simulink model "eCS_Algo_Simulation_2015b"  (R2015b)
settings: Solver=ode1  StartTime=0.0  StopTime=3  FixedStep=1/80000  RelTol=1e-3
PreLoadFcn:
  | if exist('tl_preloadfcn','file'), tl_preloadfcn(gcs,402); end
PostLoadFcn:
  | , if any(exist('dsrtsu_mdlpostloadfcn', 'file') == [2, 3, 6]), try dsrtsu_mdlpostloadfcn('Execute', bdroot); catch fprintf('Error in PostLoadFcn (dsrtsu_mdlpostloadfcn) for model "%s":\n %s\n', bdroot, lasterr); end, end,
  | if exist('tl_postloadfcn','file'), tl_postloadfcn(gcs,402); end
InitFcn:
  | Omegan=1.3024e+03;
  | xi=0.9; %0.48
  | K=0.1931;
  | K1=0.0198;
  | TauLocked=0.00255;
  | TauUnLocked=0.0042;
  | Kp=1/(2*K1);
  | Ki=Kp/((TauLocked+TauUnLocked)/2);
  | if exist('tlds_init','file'), tlds_init(gcs); end
StartFcn:
  | if exist('tlds_start','file'), tlds_start(gcs); end
StopFcn:
  | if exist('tlds_stop','file'), tlds_stop(gcs); end
model workspace (MAT data in the model file):
  au8PrevExecProfile = [0 0 0 0 0 0]
values from neighbouring files (symbols this model uses):
  AccSensor = 5    [Parameter_eCS_Algo.m]
  AlgoType = 0    [Parameter_eCS_Algo.m]
  Cxy = 1*0.017    (= 0.017)    [Acc_Init_SelV1.m]
  Cxz = 1*0.017    (= 0.017)    [Acc_Init_SelV1.m]
  Cyx = 1*0.017    (= 0.017)    [Acc_Init_SelV1.m]
  Cyz = 1*0.017    (= 0.017)    [Acc_Init_SelV1.m]
  Czx = 1*0.017    (= 0.017)    [Acc_Init_SelV1.m]
  Czy = 1*0.017    (= 0.017)    [Acc_Init_SelV1.m]
  Forced_Oscillation = 0    [Parameter_eCS_Algo.m]    (also in run_Rotation_sim.m = run)
  FreqTemperature = 10    [Acc_Init_SelV1.m]
  MaxSensorOffset = 0.3    [Acc_Init_SelV1.m]
  Mean_x_noise = 4e-3    (= 0.004)    [Acc_Init_SelV1.m]
  Mean_y_noise = 4e-3    (= 0.004)    [Acc_Init_SelV1.m]
  Mean_z_noise = 4e-3    (= 0.004)    [Acc_Init_SelV1.m]
  ODR = 8000    [Acc_Init_SelV1.m]
  offsetcorrection_on_off = 0    [Parameter_eCS_Algo.m]
  phi_pulse_rotation = 0    [Parameter_eCS_Algo.m]    (also in run_Rotation_sim.m = angle)
  pulsetype = 2    [Parameter_eCS_Algo.m]    (also in run_simulation.m = j; run_simulation_ActiveX.m = j)
  Range = 4    [Acc_Init_SelV1.m]
  sensitivity_optimisation = 0    [Parameter_eCS_Algo.m]
  TempBias = 0    [Acc_Init_SelV1.m]
  TemperatureAmp = 0    [Acc_Init_SelV1.m]
  Var_x_noise = 1.84e-9    (= 1.84e-09)    [Acc_Init_SelV1.m]
  Var_y_noise = 2.025e-09    [Acc_Init_SelV1.m]
  Var_z_noise = 1.374e-09    [Acc_Init_SelV1.m]
  w_x = 2*pi*F_x    (= 376.991118431)    [Acc_Init_SelV1.m]
  w_y = 2*pi*F_y    (= 376.991118431)    [Acc_Init_SelV1.m]
  w_z = 2*pi*F_z    (= 376.991118431)    [Acc_Init_SelV1.m]
  x_max_temp_drift = 0.061    [Acc_Init_SelV1.m]
  x_offset_enable = 0    [Acc_Init_SelV1.m]
  x_run_to_run_drift = 0.0    (= 0)    [Acc_Init_SelV1.m]
  x_temp_co_drift = 0.000    (= 0)    [Acc_Init_SelV1.m]
  Xi_x = 0.7    [Acc_Init_SelV1.m]
  Xi_y = 0.7    [Acc_Init_SelV1.m]
  Xi_z = 0.7    [Acc_Init_SelV1.m]
  y_max_temp_drift = 0.061    [Acc_Init_SelV1.m]
  y_offset_enable = 0    [Acc_Init_SelV1.m]
  y_run_to_run_drift = 0.0    (= 0)    [Acc_Init_SelV1.m]
  y_temp_co_drift = 0.000    (= 0)    [Acc_Init_SelV1.m]
  z_max_temp_drift = 0.13    [Acc_Init_SelV1.m]
  z_offset_enable = 0    [Acc_Init_SelV1.m]
  z_run_to_run_drift = 0.0    (= 0)    [Acc_Init_SelV1.m]
  z_temp_co_drift = 0.000    (= 0)    [Acc_Init_SelV1.m]
undefined symbols (not defined in the file or in its folder): controller_sample_rate, ddv, DiscIntNeverNeededParam, gmw_roada_x__m_s__, gmw_roada_y__m_s__, gmw_roadtime_2kHz, KSF_50_a_x, KSF_50_a_y, KSF_50_time, KSG_30_a_x, KSG_30_a_y, KSG_30_time, Meldorf_HindenburgstraAcceleration_x__m_s_2_, Meldorf_HindenburgstraAcceleration_y__m_s_2_, Meldorf_HindenburgstraAcceleration_z__m_s_2_, Meldorf_HindenburgstraTime__s_, pulse_FF27, pulse_MPDB, pulse_ODB40, pulse_ODB64, pulse_USNCAP, pulsetime_FF27, pulsetime_MPDB, pulsetime_ODB40, pulsetime_ODB64, pulsetime_USNCAP, Rauasphalt_60_a_x, Rauasphalt_60_a_y, Rauasphalt_60_time, sigbuilder_block, VW_416_2kHza_x_2kHz, VW_416_2kHza_y_2kHz, VW_416_2kHztime_2kHz
libraries: simulink x29, tllib x23, tl_autosar_lib x15, simulink_extras x7, LIB_TF_G_111 x2, LIB_TF_G_12_StepControl x2, LIB_TF_G_112 x1, dspsigops x1
(part 6 of 13)

== system eCS_Algo_Simulation_2015b/SAD/Subsystem/SAD/SAD/SAD_Init/For ==
  Assignment : Assignment  IndexMode=Zero-based  IndexOptions=Index vector (port)  Indices=1  OutputSizes=1  mask(TL_Assignment){data={'insideiteratedsystem',logical(1),'omitinitializations',1,'output',{'variable','SAD/Vars/au8FollowingCycle','inheritscaling',0},'date',738430.41690026619}}
      settings: CopyFcn=if exist('tl_reset_reviewflag') == 2, tl_reset_reviewflag(gcbh); end  DeleteFcn=if exist('delete_tlblock','file')==2,delete_tlblock(gcbh);end  NameChangeFcn=if exist('rename_tlblock','file')==2,rename_tlblock(gcbh);end  OpenFcn=if exist('tl_open_blockdlg','file')==2,tl_open_blockdlg(gcbh);else,open_system(gcbh,'parameter');end
      mask Help: eval(['if exist(''tl_online_help'',''file'') == 2, tl_online_help(''Topic'',''TL_Assignment''),else, web([''jar:file:///'',matlabroot,''/help/toolbox/simulink/help.jar!/slref/' lower(get_param(gcbh,'Blocktype')) '.html''], ''-helpbrowser''),end'])
      mask Display: plot([-0.1, 1.05, NaN, -0.1, 1.05],[.01, .01, NaN, .99, .99]);
  BusCreator : BusCreator  Inputs=2
  Constant : Constant  Value=[255 255 255 255]  mask(TL_Constant){data={'date',738430.41690041672}}
      settings: CopyFcn=if exist('tl_reset_reviewflag','file')==2,tl_reset_reviewflag(gcbh);end  DeleteFcn=if exist('delete_tlblock','file')==2,delete_tlblock(gcbh);end  NameChangeFcn=if exist('rename_tlblock','file')==2,rename_tlblock(gcbh);end  OpenFcn=if exist('tl_open_blockdlg','file')==2,tl_open_blockdlg(gcbh);else,open_system(gcbh,'parameter');end
      mask Help: eval(['if exist(''tl_online_help'',''file'') == 2, tl_online_help(''Topic'',''TL_Constant''),else, web([''jar:file:///'',matlabroot,''/help/toolbox/simulink/help.jar!/slref/' lower(get_param(gcbh,'Blocktype')) '.html''], ''-helpbrowser''),end'])
      mask Display: plot([-0.1, 1.05, NaN, -0.1, 1.05],[.01, .01, NaN, .99, .99]);
  Constant1 : Constant  Value=ddv('SAD/Macros/Profiles/KU8_PROFILE_SIZE')  mask(TL_Constant){data={'output',{'variable','SAD/Macros/Profiles/KU8_PROFILE_SIZE'},'date',738430.41690053244}}
      settings: CopyFcn=if exist('tl_reset_reviewflag','file')==2,tl_reset_reviewflag(gcbh);end  DeleteFcn=if exist('delete_tlblock','file')==2,delete_tlblock(gcbh);end  NameChangeFcn=if exist('rename_tlblock','file')==2,rename_tlblock(gcbh);end  OpenFcn=if exist('tl_open_blockdlg','file')==2,tl_open_blockdlg(gcbh);else,open_system(gcbh,'parameter');end
      mask Help: eval(['if exist(''tl_online_help'',''file'') == 2, tl_online_help(''Topic'',''TL_Constant''),else, web([''jar:file:///'',matlabroot,''/help/toolbox/simulink/help.jar!/slref/' lower(get_param(gcbh,'Blocktype')) '.html''], ''-helpbrowser''),end'])
      mask Display: plot([-0.1, 1.05, NaN, -0.1, 1.05],[.01, .01, NaN, .99, .99]);
  Constant2 : Constant  Value=[255 255 255 255]  mask(TL_Constant){data={'date',738430.41690065968}}
      settings: CopyFcn=if exist('tl_reset_reviewflag','file')==2,tl_reset_reviewflag(gcbh);end  DeleteFcn=if exist('delete_tlblock','file')==2,delete_tlblock(gcbh);end  NameChangeFcn=if exist('rename_tlblock','file')==2,rename_tlblock(gcbh);end  OpenFcn=if exist('tl_open_blockdlg','file')==2,tl_open_blockdlg(gcbh);else,open_system(gcbh,'parameter');end
      mask Help: eval(['if exist(''tl_online_help'',''file'') == 2, tl_online_help(''Topic'',''TL_Constant''),else, web([''jar:file:///'',matlabroot,''/help/toolbox/simulink/help.jar!/slref/' lower(get_param(gcbh,'Blocktype')) '.html''], ''-helpbrowser''),end'])
      mask Display: plot([-0.1, 1.05, NaN, -0.1, 1.05],[.01, .01, NaN, .99, .99]);
  Constant3 : Constant  Value=ddv('Common/KU8_THREE')  mask(TL_Constant){data={'output',{'variable','Common/KU8_THREE'},'date',738430.41690077551}}
      settings: CopyFcn=if exist('tl_reset_reviewflag','file')==2,tl_reset_reviewflag(gcbh);end  DeleteFcn=if exist('delete_tlblock','file')==2,delete_tlblock(gcbh);end  NameChangeFcn=if exist('rename_tlblock','file')==2,rename_tlblock(gcbh);end  OpenFcn=if exist('tl_open_blockdlg','file')==2,tl_open_blockdlg(gcbh);else,open_system(gcbh,'parameter');end
      mask Help: eval(['if exist(''tl_online_help'',''file'') == 2, tl_online_help(''Topic'',''TL_Constant''),else, web([''jar:file:///'',matlabroot,''/help/toolbox/simulink/help.jar!/slref/' lower(get_param(gcbh,'Blocktype')) '.html''], ''-helpbrowser''),end'])
      mask Display: plot([-0.1, 1.05, NaN, -0.1, 1.05],[.01, .01, NaN, .99, .99]);
  Constant4 : Constant  Value=ddv('SAD/NVP/Profiles/CFG_au8ProfileLib')  mask(TL_Constant){data={'output',{'variable','SAD/NVP/Profiles/CFG_au8ProfileLib'},'date',738430.41690089123}}
      settings: CopyFcn=if exist('tl_reset_reviewflag','file')==2,tl_reset_reviewflag(gcbh);end  DeleteFcn=if exist('delete_tlblock','file')==2,delete_tlblock(gcbh);end  NameChangeFcn=if exist('rename_tlblock','file')==2,rename_tlblock(gcbh);end  OpenFcn=if exist('tl_open_blockdlg','file')==2,tl_open_blockdlg(gcbh);else,open_system(gcbh,'parameter');end
      mask Help: eval(['if exist(''tl_online_help'',''file'') == 2, tl_online_help(''Topic'',''TL_Constant''),else, web([''jar:file:///'',matlabroot,''/help/toolbox/simulink/help.jar!/slref/' lower(get_param(gcbh,'Blocktype')) '.html''], ''-helpbrowser''),end'])
      mask Display: plot([-0.1, 1.05, NaN, -0.1, 1.05],[.01, .01, NaN, .99, .99]);
  Constant5 : Constant  mask(TL_Constant){data={'date',738430.41690100695}}
      settings: CopyFcn=if exist('tl_reset_reviewflag') == 2, tl_reset_reviewflag(gcbh); end  DeleteFcn=if exist('delete_tlblock','file')==2,delete_tlblock(gcbh);end  NameChangeFcn=if exist('rename_tlblock','file')==2,rename_tlblock(gcbh);end  OpenFcn=if exist('tl_open_blockdlg','file')==2,tl_open_blockdlg(gcbh);else,open_system(gcbh,'parameter');end
      mask Help: eval(['if exist(''tl_online_help'',''file'') == 2, tl_online_help(''Topic'',''TL_Constant''),else, web([''jar:file:///'',matlabroot,''/help/toolbox/simulink/help.jar!/slref/' lower(get_param(gcbh,'Blocktype')) '.html''], ''-helpbrowser''),end'])
      mask Display: plot([-0.1, 1.05, NaN, -0.1, 1.05],[.01, .01, NaN, .99, .99]);
  FollowingCycle : Selector  IndexMode=Zero-based  IndexOptions=Index vector (port)  Indices=[1 3]  OutputSizes=1
  For Iterator : ForIterator  IterationLimit=4  IndexMode=Zero-based  IterationVariableDataType=int8
  Product1 : Product  Inputs=**  RndMeth=Zero  mask(TL_Product){data={'output',{'type','UInt16'},'date',738430.41690100695}}
      settings: CopyFcn=if exist('tl_reset_reviewflag') == 2, tl_reset_reviewflag(gcbh); end  DeleteFcn=if exist('delete_tlblock','file')==2,delete_tlblock(gcbh);end  NameChangeFcn=if exist('rename_tlblock','file')==2,rename_tlblock(gcbh);end  OpenFcn=if exist('tl_open_blockdlg','file')==2,tl_open_blockdlg(gcbh);else,open_system(gcbh,'parameter');end
      mask Help: eval(['if exist(''tl_online_help'',''file'') == 2, tl_online_help(''Topic'',''TL_Product''),else, web([''jar:file:///'',matlabroot,''/help/toolbox/simulink/help.jar!/slref/' lower(get_param(gcbh,'Blocktype')) '.html''], ''-helpbrowser''),end'])
      mask Display: plot([-0.1, 1.05, NaN, -0.1, 1.05],[.01, .01, NaN, .99, .99]);
  Rescaler : DataTypeConversion  mask(TL_Rescaler){data={'output',{'type','UInt8'},'date',738430.4169011343}}
      settings: DeleteFcn=if exist('delete_tlblock','file')==2,delete_tlblock(gcbh);end  NameChangeFcn=if exist('rename_tlblock','file')==2,rename_tlblock(gcbh);end  OpenFcn=if exist('tl_open_blockdlg','file')==2,tl_open_blockdlg(gcbh);else,open_system(gcbh,'parameter');end
      mask Help: eval(['if exist(''tl_online_help'',''file'') == 2, tl_online_help(''Topic'',''TL_Rescaler''),else, web([''jar:file:///'',matlabroot,''/help/toolbox/simulink/help.jar!/slref/' lower(get_param(gcbh,'Blocktype')) '.html''], ''-helpbrowser''),end'])
      mask Display: plot([-0.1, 1.05, NaN, -0.1, 1.05],[.01, .01, NaN, .99, .99]);
  Rescaler1 : DataTypeConversion  mask(TL_Rescaler){data={'output',{'type','UInt8'},'date',738430.41690125002}}
      settings: DeleteFcn=if exist('delete_tlblock','file')==2,delete_tlblock(gcbh);end  NameChangeFcn=if exist('rename_tlblock','file')==2,rename_tlblock(gcbh);end  OpenFcn=if exist('tl_open_blockdlg','file')==2,tl_open_blockdlg(gcbh);else,open_system(gcbh,'parameter');end
      mask Help: eval(['if exist(''tl_online_help'',''file'') == 2, tl_online_help(''Topic'',''TL_Rescaler''),else, web([''jar:file:///'',matlabroot,''/help/toolbox/simulink/help.jar!/slref/' lower(get_param(gcbh,'Blocktype')) '.html''], ''-helpbrowser''),end'])
      mask Display: plot([-0.1, 1.05, NaN, -0.1, 1.05],[.01, .01, NaN, .99, .99]);
  Sum : Sum  mask(TL_Sum){data={'output',{'type','UInt16'},'date',738430.41690136574}}
      settings: CopyFcn=if exist('tl_reset_reviewflag') == 2, tl_reset_reviewflag(gcbh); end  DeleteFcn=if exist('delete_tlblock','file')==2,delete_tlblock(gcbh);end  NameChangeFcn=if exist('rename_tlblock','file')==2,rename_tlblock(gcbh);end  OpenFcn=if exist('tl_open_blockdlg','file')==2,tl_open_blockdlg(gcbh);else,open_system(gcbh,'parameter');end
      mask Help: eval(['if exist(''tl_online_help'',''file'') == 2, tl_online_help(''Topic'',''TL_Sum''),else, web([''jar:file:///'',matlabroot,''/help/toolbox/simulink/help.jar!/slref/' lower(get_param(gcbh,'Blocktype')) '.html''], ''-helpbrowser''),end'])
      mask Display: plot([-0.1, 1.05, NaN, -0.1, 1.05],[.01, .01, NaN, .99, .99]);
  Sum2 : Sum  Inputs=+-  mask(TL_Sum){data={'output',{'type','UInt8'},'date',738430.41690148145}}
      settings: CopyFcn=if exist('tl_reset_reviewflag') == 2, tl_reset_reviewflag(gcbh); end  DeleteFcn=if exist('delete_tlblock','file')==2,delete_tlblock(gcbh);end  NameChangeFcn=if exist('rename_tlblock','file')==2,rename_tlblock(gcbh);end  OpenFcn=if exist('tl_open_blockdlg','file')==2,tl_open_blockdlg(gcbh);else,open_system(gcbh,'parameter');end
      mask Help: eval(['if exist(''tl_online_help'',''file'') == 2, tl_online_help(''Topic'',''TL_Sum''),else, web([''jar:file:///'',matlabroot,''/help/toolbox/simulink/help.jar!/slref/' lower(get_param(gcbh,'Blocktype')) '.html''], ''-helpbrowser''),end'])
      mask Display: plot([-0.1, 1.05, NaN, -0.1, 1.05],[.01, .01, NaN, .99, .99]);
  Switch : Switch  Criteria=u2 ~= 0  mask(TL_Switch){data={'output',{'type','UInt8'},'date',738430.41690159717}}
      settings: CopyFcn=if exist('tl_reset_reviewflag') == 2, tl_reset_reviewflag(gcbh); end  DeleteFcn=if exist('delete_tlblock','file')==2,delete_tlblock(gcbh);end  NameChangeFcn=if exist('rename_tlblock','file')==2,rename_tlblock(gcbh);end  OpenFcn=if exist('tl_open_blockdlg','file')==2,tl_open_blockdlg(gcbh);else,open_system(gcbh,'parameter');end
      mask Help: eval(['if exist(''tl_online_help'',''file'') == 2, tl_online_help(''Topic'',''TL_Switch''),else, web([''jar:file:///'',matlabroot,''/help/toolbox/simulink/help.jar!/slref/' lower(get_param(gcbh,'Blocktype')) '.html''], ''-helpbrowser''),end'])
      mask Display: plot([-0.1, 1.05, NaN, -0.1, 1.05],[.01, .01, NaN, .99, .99]);
  While Iterator Subsystem : Subsystem  TreatAsAtomicUnit=on
  au8LastStepIdx : Assignment  IndexMode=Zero-based  IndexOptions=Index vector (port)  Indices=1  OutputSizes=1  mask(TL_Assignment){data={'insideiteratedsystem',logical(1),'omitinitializations',1,'output',{'variable','SAD/Vars/au8LastStepidx','inheritscaling',0},'date',738430.41690241895}}
      settings: CopyFcn=if exist('tl_reset_reviewflag') == 2, tl_reset_reviewflag(gcbh); end  DeleteFcn=if exist('delete_tlblock','file')==2,delete_tlblock(gcbh);end  NameChangeFcn=if exist('rename_tlblock','file')==2,rename_tlblock(gcbh);end  OpenFcn=if exist('tl_open_blockdlg','file')==2,tl_open_blockdlg(gcbh);else,open_system(gcbh,'parameter');end
      mask Help: eval(['if exist(''tl_online_help'',''file'') == 2, tl_online_help(''Topic'',''TL_Assignment''),else, web([''jar:file:///'',matlabroot,''/help/toolbox/simulink/help.jar!/slref/' lower(get_param(gcbh,'Blocktype')) '.html''], ''-helpbrowser''),end'])
      mask Display: plot([-0.1, 1.05, NaN, -0.1, 1.05],[.01, .01, NaN, .99, .99]);
  stProfileCfg : Outport
  wires:
  Constant1/1 -> Product1/2
  Constant4/1 -> FollowingCycle/1
  For Iterator/1 -> au8LastStepIdx/3, Assignment/3, Product1/1
  Product1/1 -> While Iterator Subsystem/1(ProfileOffset), Sum/1
  Constant3/1 -> Sum/2
  Sum/1 -> FollowingCycle/2
  FollowingCycle/1 -> Rescaler/1
  Constant/1 -> Assignment/1
  Rescaler/1 -> Assignment/2
  au8LastStepIdx/1 -> BusCreator/2  "au8LastStep"
  BusCreator/1 -> stProfileCfg/1  "stProfileCfg"
  Assignment/1 -> BusCreator/1  "au8FollowingProfile"
  Rescaler1/1 -> au8LastStepIdx/2
  Constant2/1 -> au8LastStepIdx/1
  While Iterator Subsystem/1(LastStepIdx) -> Sum2/1, Switch/3, Switch/2
  Switch/1 -> Rescaler1/1
  Sum2/1 -> Switch/1
  Constant5/1 -> Sum2/2

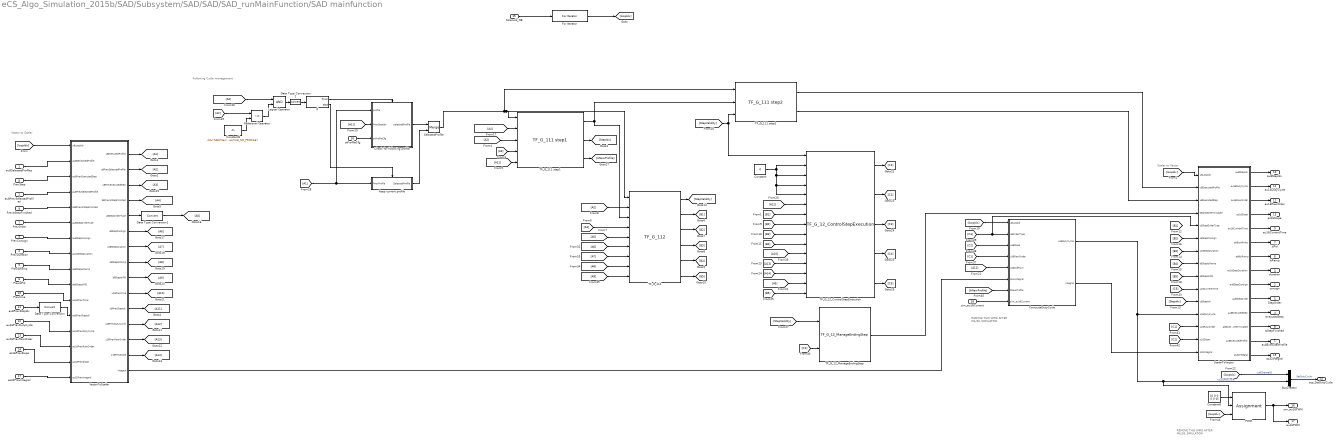
== system eCS_Algo_Simulation_2015b/SAD/Subsystem/SAD/SAD/SAD_runMainFunction/SAD mainfunction ==
  note: REMOVE THIS WIRE AFTER
      | MIL/SIL SIMULATION
  note: Scalar to Vector
  note: Vector to Scalar
  note: Following Cycle management
  note: REMOVE THIS WIRE AFTER
      | MIL/SIL SIMULATION
  au8SelectedProfiles : Inport
  au8PrevSelectedProfiles : Inport  Port=2
  PrevConsign : Inport  Port=3
  PrevDuration : Inport  Port=4
  PrevIsRamp : Inport  Port=5
  PrevIsPid : Inport  Port=6
  PrevOrder : Inport  Port=7
  PrevStep : Inport  Port=8
  PrevIsStepFinished : Inport  Port=9
  Prevtime : Inport  Port=10
  au8PrevStepIdx : Inport  Port=11
  au16PrevDutyCycle : Inport  Port=12
  au16PrevRawOrder : Inport  Port=13
  as16PrevSlope : Inport  Port=14
  Solenoid_NB : Inport  Port=15
  stProfileCfg : Inport  Port=16
  as32PrevIntegral : Inport  Port=17
  sim_au16Current : Inport  Port=18  PortDimensions=6  mask(TL_Inport){data={'output',{'type','UInt16'},'autosar',{'useautosarcommunication',1,'senderreceiverport','prrSolenoidCurrent','dataelement','au16Current'},'date',738433.42446635419}}
      settings: CopyFcn=if exist('tl_reset_reviewflag','file')==2,tl_reset_reviewflag(gcbh);end  DeleteFcn=if exist('delete_tlblock','file')==2,delete_tlblock(gcbh);end  NameChangeFcn=if exist('rename_tlblock','file')==2,rename_tlblock(gcbh);end  OpenFcn=if exist('tl_open_blockdlg','file')==2,tl_open_blockdlg(gcbh);else,open_system(gcbh,'parameter');end
      mask Help: eval(['if exist(''tl_online_help'',''file'') == 2, tl_online_help(''Topic'',''TL_Inport''),else, web([''jar:file:///'',matlabroot,''/help/toolbox/simulink/help.jar!/slref/' lower(get_param(gcbh,'Blocktype')) '.html''], ''-helpbrowser''),end'])
      mask Display: plot([0.2 0.35 NaN 0.65 0.8],[0 1 NaN 0 1]);
  BusCreator : BusCreator  Inputs=2
  Check for following profile : Subsystem  TreatAsAtomicUnit=on
  ComputeDutyCycle : Subsystem
  Constant : Constant  Value=0  mask(TL_Constant){data={'date',738430.41690910875}}
      settings: CopyFcn=if exist('tl_reset_reviewflag') == 2, tl_reset_reviewflag(gcbh); end  DeleteFcn=if exist('delete_tlblock','file')==2,delete_tlblock(gcbh);end  NameChangeFcn=if exist('rename_tlblock','file')==2,rename_tlblock(gcbh);end  OpenFcn=if exist('tl_open_blockdlg','file')==2,tl_open_blockdlg(gcbh);else,open_system(gcbh,'parameter');end
      mask Help: eval(['if exist(''tl_online_help'',''file'') == 2, tl_online_help(''Topic'',''TL_Constant''),else, web([''jar:file:///'',matlabroot,''/help/toolbox/simulink/help.jar!/slref/' lower(get_param(gcbh,'Blocktype')) '.html''], ''-helpbrowser''),end'])
      mask Display: plot([-0.1, 1.05, NaN, -0.1, 1.05],[.01, .01, NaN, .99, .99]);
  Constant6 : Constant  Value=[0 0 0 0 0 0]  mask(TL_Constant){data={'date',738430.41691166663}}
      settings: CopyFcn=if exist('tl_reset_reviewflag') == 2, tl_reset_reviewflag(gcbh); end  DeleteFcn=if exist('delete_tlblock','file')==2,delete_tlblock(gcbh);end  NameChangeFcn=if exist('rename_tlblock','file')==2,rename_tlblock(gcbh);end  OpenFcn=if exist('tl_open_blockdlg','file')==2,tl_open_blockdlg(gcbh);else,open_system(gcbh,'parameter');end
      mask Help: eval(['if exist(''tl_online_help'',''file'') == 2, tl_online_help(''Topic'',''TL_Constant''),else, web([''jar:file:///'',matlabroot,''/help/toolbox/simulink/help.jar!/slref/' lower(get_param(gcbh,'Blocktype')) '.html''], ''-helpbrowser''),end'])
      mask Display: plot([-0.1, 1.05, NaN, -0.1, 1.05],[.01, .01, NaN, .99, .99]);
  Constant8 : Constant  Value=ddv('SAD/Macros/Profiles/KU8_NO_PROFILE')  mask(TL_Constant){data={'output',{'variable','SAD/Macros/Profiles/KU8_NO_PROFILE'},'date',738430.41690531245}}
      settings: CopyFcn=if exist('tl_reset_reviewflag','file')==2,tl_reset_reviewflag(gcbh);end  DeleteFcn=if exist('delete_tlblock','file')==2,delete_tlblock(gcbh);end  NameChangeFcn=if exist('rename_tlblock','file')==2,rename_tlblock(gcbh);end  OpenFcn=if exist('tl_open_blockdlg','file')==2,tl_open_blockdlg(gcbh);else,open_system(gcbh,'parameter');end
      mask Help: eval(['if exist(''tl_online_help'',''file'') == 2, tl_online_help(''Topic'',''TL_Constant''),else, web([''jar:file:///'',matlabroot,''/help/toolbox/simulink/help.jar!/slref/' lower(get_param(gcbh,'Blocktype')) '.html''], ''-helpbrowser''),end'])
      mask Display: plot([-0.1, 1.05, NaN, -0.1, 1.05],[.01, .01, NaN, .99, .99]);
  Data Type Conversion : DataTypeConversion
  Data Type Conversion1 : DataTypeConversion
  Data Type Conversion2 : DataTypeConversion
  For Iterator : ForIterator  IterationSource=external  IterationLimit=6  IndexMode=Zero-based  IterationVariableDataType=int8
  If : If  IfExpression=u1
  Keep current profile : Subsystem  TreatAsAtomicUnit=on
  Logical Operator : Logic  AllPortsSameDT=off  OutDataTypeStr=boolean  mask(TL_LogicalOperator){data={'date',738598.66698877316}}
      settings: DeleteFcn=if exist('delete_tlblock','file')==2,delete_tlblock(gcbh);end  NameChangeFcn=if exist('rename_tlblock','file')==2,rename_tlblock(gcbh);end  OpenFcn=if exist('tl_open_blockdlg','file')==2,tl_open_blockdlg(gcbh);else,open_system(gcbh,'parameter');end
      mask Help: eval(['if exist(''tl_online_help'',''file'') == 2, tl_online_help(''Topic'',''TL_LogicalOperator''),else, web([''jar:file:///'',matlabroot,''/help/toolbox/simulink/help.jar!/slref/' lower(get_param(gcbh,'Blocktype')) '.html''], ''-helpbrowser''),end'])
      mask Display: plot([-0.1, 1.05, NaN, -0.1, 1.05],[.01, .01, NaN, .99, .99]);
  PWM : Assignment  IndexMode=Zero-based  IndexOptions=Index vector (port)  Indices=1  OutputSizes=1  mask(TL_Assignment){data={'insideiteratedsystem',logical(1),'omitinitializations',1,'output',{'description',['Resolution:  2^-15'],'name','$D','max',[32768 32767 32767 32767 32767 32767],'min',[0 -32768 -32768 -32768 -32768 -32768],'type','UInt16','scaling','VOID_SCALING','inheritscaling',0},'date',738496.36831776623}}
      settings: CopyFcn=if exist('tl_reset_reviewflag') == 2, tl_reset_reviewflag(gcbh); end  DeleteFcn=if exist('delete_tlblock','file')==2,delete_tlblock(gcbh);end  NameChangeFcn=if exist('rename_tlblock','file')==2,rename_tlblock(gcbh);end  OpenFcn=if exist('tl_open_blockdlg','file')==2,tl_open_blockdlg(gcbh);else,open_system(gcbh,'parameter');end
      mask Help: eval(['if exist(''tl_online_help'',''file'') == 2, tl_online_help(''Topic'',''TL_Assignment''),else, web([''jar:file:///'',matlabroot,''/help/toolbox/simulink/help.jar!/slref/' lower(get_param(gcbh,'Blocktype')) '.html''], ''-helpbrowser''),end'])
      mask Display: plot([-0.1, 1.05, NaN, -0.1, 1.05],[.01, .01, NaN, .99, .99]);
  Relational Operator : RelationalOperator  Operator=~=  OutDataTypeStr=boolean  mask(TL_RelationalOperator){data={'date',738598.66684523143}}
      settings: DeleteFcn=if exist('delete_tlblock','file')==2,delete_tlblock(gcbh);end  NameChangeFcn=if exist('rename_tlblock','file')==2,rename_tlblock(gcbh);end  OpenFcn=if exist('tl_open_blockdlg','file')==2,tl_open_blockdlg(gcbh);else,open_system(gcbh,'parameter');end
      mask Help: eval(['if exist(''tl_online_help'',''file'') == 2, tl_online_help(''Topic'',''TL_RelationalOperator''),else, web([''jar:file:///'',matlabroot,''/help/toolbox/simulink/help.jar!/slref/' lower(get_param(gcbh,'Blocktype')) '.html''], ''-helpbrowser''),end'])
      mask Display: plot([-0.1, 1.05, NaN, -0.1, 1.05],[.01, .01, NaN, .99, .99]);
  ScalarToVector : Subsystem  TreatAsAtomicUnit=on
  SelectedProfile : Merge  mask(TL_Merge){data={'date',738430.41691454861}}
      settings: CopyFcn=if exist('tl_reset_reviewflag') == 2, tl_reset_reviewflag(gcbh); end  DeleteFcn=if exist('delete_tlblock','file')==2,delete_tlblock(gcbh);end  NameChangeFcn=if exist('rename_tlblock','file')==2,rename_tlblock(gcbh);end  OpenFcn=if exist('tl_open_blockdlg','file')==2,tl_open_blockdlg(gcbh);else,open_system(gcbh,'parameter');end
      mask Help: eval(['if exist(''tl_online_help'',''file'') == 2, tl_online_help(''Topic'',''TL_Merge''),else, web([''jar:file:///'',matlabroot,''/help/toolbox/simulink/help.jar!/slref/' lower(get_param(gcbh,'Blocktype')) '.html''], ''-helpbrowser''),end'])
      mask Display: plot([-0.1, 1.05, NaN, -0.1, 1.05],[.01, .01, NaN, .99, .99]);
  TF_G_111 step1 : LIB_TF_G_111/TF_G_111 step1
  TF_G_111 step2 : LIB_TF_G_111/TF_G_111 step2  Description=The subsystemDetermineExecutedFunction block is in charge of providing the current executed function output.
  TF_G_112 : LIB_TF_G_112/TF_G_112
  TF_G_12_ControlStepExecution : LIB_TF_G_12_StepControl/TF_G_12_ControlStepExecution
  TF_G_12_ManageEndingStep : LIB_TF_G_12_StepControl/TF_G_12_ManageEndingStep
  VectorToScalar : Subsystem  TreatAsAtomicUnit=on
      settings: MinAlgLoopOccurrences=on
  au8ExecutedProfile : Outport
  consign : Outport  Port=2
  duration : Outport  Port=3
  executedStep : Outport  Port=4
  StepOrder : Outport  Port=5
  IsRamp : Outport  Port=6
  IsPid : Outport  Port=7
  IsStepFinished : Outport  Port=8
  au16CurrentTime : Outport  Port=9
  au8StepIdx : Outport  Port=10
  au16DutyCycle : Outport  Port=11
  au16RawOrder : Outport  Port=12
  as16Slope : Outport  Port=13
  scp_SetDutyCycle : Outport  Port=14  mask(TL_BusOutport){data={'#autoscaling',2,'#message',2,'#output',2,'#logdata',2,'signals',{{'SetDutyCycle',{'cu8ChannelID';'cu16DutyCycle'}}},'autosar',{'useautosarcommunication',1,'kind',4,'clientserverport','pclPwmServices','operation','SetDutyCycle'},'date',738496.45470876154}}
      settings: CopyFcn=if exist('tl_reset_reviewflag') == 2, tl_reset_reviewflag(gcbh); end  DeleteFcn=if exist('delete_tlblock','file')==2,delete_tlblock(gcbh);end  NameChangeFcn=if exist('rename_tlblock','file')==2,rename_tlblock(gcbh);end  OpenFcn=if exist('tl_open_blockdlg','file')==2,tl_open_blockdlg(gcbh);else,open_system(gcbh,'parameter');end
      mask Help: eval(['if exist(''tl_online_help'',''file'') == 2, tl_online_help(''Topic'',''TL_Outport''),else, web([''jar:file:///'',matlabroot,''/help/toolbox/simulink/help.jar!/slref/' lower(get_param(gcbh,'Blocktype')) '.html''], ''-helpbrowser''),end'])
      mask Display: plot([0.2 0.35 NaN 0.65 0.8],[0 1 NaN 0 1]);
  as32Integral : Outport  Port=15
  sim_au16PWM : Outport  Port=16  PortDimensions=6  mask(TL_Outport){data={'output',{'type','UInt16'},'autosar',{'useautosarcommunication',1,'senderreceiverport','sim_psrSolenoidPWM','dataelement','au16Pwm'},'date',738591.6796040741}}
      settings: CopyFcn=if exist('tl_reset_reviewflag','file')==2,tl_reset_reviewflag(gcbh);end  DeleteFcn=if exist('delete_tlblock','file')==2,delete_tlblock(gcbh);end  NameChangeFcn=if exist('rename_tlblock','file')==2,rename_tlblock(gcbh);end  OpenFcn=if exist('tl_open_blockdlg','file')==2,tl_open_blockdlg(gcbh);else,open_system(gcbh,'parameter');end
      mask Help: eval(['if exist(''tl_online_help'',''file'') == 2, tl_online_help(''Topic'',''TL_Outport''),else, web([''jar:file:///'',matlabroot,''/help/toolbox/simulink/help.jar!/slref/' lower(get_param(gcbh,'Blocktype')) '.html''], ''-helpbrowser''),end'])
      mask Display: plot([0.2 0.35 NaN 0.65 0.8],[0 1 NaN 0 1]);
  au16PWM : Outport  Port=17
  wires:
  For Iterator/1 -> [loopIdx]
  au8SelectedProfiles/1 -> VectorToScalar/2(au8SeclectedProfile)
  [loopIdx] -> VectorToScalar/1(u8LoopIdx)
  VectorToScalar/1(u8ExecutedProfile) -> [A1]
  VectorToScalar/2(u8PrevSelectedProfile) -> [A2]
  [A2] -> TF_G_111 step1/3
  TF_G_111 step1/1 -> TF_G_112/3, TF_G_111 step2/2
  [A2] -> TF_G_112/2
  [A4] -> TF_G_111 step1/2
  [loopIdx] -> ScalarToVector/1(u8LoopIdx)
  TF_G_111 step2/1 -> ScalarToVector/2(u8ExecutedProfile)
  TF_G_12_ManageEndingStep/1 -> ScalarToVector/4(b8IsStepTerminated)
  TF_G_111 step2/2 -> ScalarToVector/3(u8ExecutedStep)
  TF_G_112/2 -> [B1]
  TF_G_112/3 -> [B2]
  TF_G_112/4 -> [B3]
  TF_G_112/5 -> [B4]
  TF_G_112/6 -> [B5]
  [B3] -> TF_G_12_ControlStepExecution/9
  [B4] -> TF_G_12_ControlStepExecution/10
  [B2] -> ScalarToVector/6(u8StepConsign)
  [B4] -> ScalarToVector/8(b8StepIsRamp)
  [B3] -> ScalarToVector/7(u16StepDuration)
  [B5] -> ScalarToVector/9(b8StepIsPID)
  VectorToScalar/5(u8StepOrderType) -> Data Type Conversion1/1
  VectorToScalar/4(b8PrevIsStepFinished) -> [A4]
  Constant/1 -> TF_G_12_ControlStepExecution/2, TF_G_12_ControlStepExecution/5, TF_G_12_ControlStepExecution/4, TF_G_12_ControlStepExecution/3
  PrevConsign/1 -> VectorToScalar/7(au8StepConsign)
  PrevDuration/1 -> VectorToScalar/8(au16StepDuration)
  PrevIsRamp/1 -> VectorToScalar/9(ab8StepIsRamp)
  PrevIsPid/1 -> VectorToScalar/10(ab8StepIsPID)
  PrevOrder/1 -> VectorToScalar/6(au8StepOrderType)
  PrevIsStepFinished/1 -> VectorToScalar/5(ab8PrevIsStepFinished)
  PrevStep/1 -> VectorToScalar/3(au8PrevExecutedStep)
  au8PrevSelectedProfiles/1 -> VectorToScalar/4(au8PrevSelectedProfile)
  Prevtime/1 -> VectorToScalar/11(au16PrevTime)
  TF_G_111 step1/2 -> [StepIdx]
  [A11] -> TF_G_111 step1/5
  [StepIdx] -> ScalarToVector/11(u8StepIdx)
  VectorToScalar/11(u8PrevStepIdx) -> [A11]
  Data Type Conversion/1 -> VectorToScalar/12(au8PrevStepIdx)
  [B2] -> TF_G_12_ControlStepExecution/8
  au16PrevDutyCycle/1 -> VectorToScalar/13(au16PrevDutyCycle)
  [loopIdx] -> ComputeDutyCycle/1(u8LoopId)
  VectorToScalar/12(u16PrevDutyCycle) -> [A12]
  [A12] -> TF_G_12_ControlStepExecution/6
  [A12] -> ComputeDutyCycle/5(u16OldPwm)
  VectorToScalar/13(u16PrevRawOrder) -> [A13]
  VectorToScalar/14(s16PrevSlope) -> [A14]
  [A13] -> TF_G_12_ControlStepExecution/12
  [A14] -> TF_G_12_ControlStepExecution/13
  [B1] -> TF_G_12_ControlStepExecution/7
  au16PrevRawOrder/1 -> VectorToScalar/14(au16PrevRawOrder)
  as16PrevSlope/1 -> VectorToScalar/15(as16PrevSlope)
  [B5] -> TF_G_12_ControlStepExecution/15
  TF_G_112/1 -> [StepValidity]
  [StepValidity] -> TF_G_12_ControlStepExecution/1, TF_G_111 step2/3
  [StepValidity] -> TF_G_12_ManageEndingStep/1
  If/1 -> Check for following profile/Action
  If/2 -> Keep current profile/Action
  Check for following profile/1(selectedProfile) -> SelectedProfile/1
  Keep current profile/1(SelectedProfile) -> SelectedProfile/2
  [A1] -> Keep current profile/1(PrevProfile), Check for following profile/1(profile)
  [A11] -> Check for following profile/2(PrevStepIdx)
  Solenoid_NB/1 -> For Iterator/1
  ScalarToVector/2(au16DutyCycle) -> au16DutyCycle/1
  ScalarToVector/3(au16RawOrder) -> au16RawOrder/1
  ScalarToVector/4(as16Slope) -> as16Slope/1
  ScalarToVector/5(au16CurrentTime) -> au16CurrentTime/1
  ScalarToVector/6(ab8IsInfinite) -> IsPid/1
  ScalarToVector/7(ab8IsRamp) -> IsRamp/1
  ScalarToVector/8(au16StepDuration) -> duration/1
  ScalarToVector/9(au8StepConsign) -> consign/1
  ScalarToVector/10(au8StepOrder) -> StepOrder/1
  ScalarToVector/11(au8ExecutedStep) -> executedStep/1
  ScalarToVector/12(ab8IsStepTerminated) -> IsStepFinished/1
  ScalarToVector/13(au8ExecutedProfile) -> au8ExecutedProfile/1
  VectorToScalar/3(u8PrevExecutedStep) -> [A3]
  [A3] -> TF_G_111 step1/4
  [A3] -> TF_G_112/4
  Data Type Conversion1/1 -> [A5]
  [A5] -> TF_G_112/5
  [A5] -> TF_G_12_ControlStepExecution/14
  VectorToScalar/6(u8StepConsign) -> [A6]
  [A6] -> TF_G_112/6
  VectorToScalar/7(u16StepDuration) -> [A7]
  [A7] -> TF_G_112/7
  VectorToScalar/8(b8StepIsRamp) -> [A8]
  [A8] -> TF_G_112/8
  VectorToScalar/9(b8StepIsPID) -> [A9]
  [A9] -> TF_G_112/9
  VectorToScalar/10(u16Prevtime) -> [A10]
  [A10] -> TF_G_12_ControlStepExecution/11
  TF_G_12_ControlStepExecution/1 -> [C1]
  [C1] -> ComputeDutyCycle/4(u16RawOrder)
  TF_G_12_ControlStepExecution/2 -> [C2]
  TF_G_12_ControlStepExecution/3 -> [C3]
  [C2] -> ComputeDutyCycle/3(u16Slope)
  [C3] -> ScalarToVector/5(u8StepOrderType), ComputeDutyCycle/2(u8OrderType)
  TF_G_12_ControlStepExecution/4 -> [C4]
  [C4] -> TF_G_12_ManageEndingStep/2
  TF_G_12_ControlStepExecution/5 -> [C5]
  [C1] -> ScalarToVector/13(u16RawOrder)
  [C2] -> ScalarToVector/14(s16Slope)
  [C5] -> ScalarToVector/10(u16CurrentTime)
  ScalarToVector/1(au8StepIdx) -> au8StepIdx/1
  au8PrevStepIdx/1 -> Data Type Conversion/1
  ComputeDutyCycle/1(u16DutyCycle) -> ScalarToVector/12(u16DutyCycle), PWM/2, BusCreator/2  "cu16DutyCycle"
  [loopIdx] -> BusCreator/1  "cu8ChannelID"
  BusCreator/1 -> scp_SetDutyCycle/1  "SetDutyCycle"
  stProfileCfg/1 -> Check for following profile/3(stProfileCfg)
  [loopIdx] -> PWM/3
  Constant6/1 -> PWM/1
  ScalarToVector/14(as32Integral) -> as32Integral/1
  ComputeDutyCycle/2(integral) -> ScalarToVector/15(s32Integral)
  as32PrevIntegral/1 -> VectorToScalar/16(as32PrevIntegral)
  VectorToScalar/15(Integral) -> ComputeDutyCycle/6(prevIntegral)
  TF_G_111 step1/3 -> [bNewProfile]
  [bNewProfile] -> ComputeDutyCycle/7(bNewProfile)
  PWM/1 -> au16PWM/1, sim_au16PWM/1
  sim_au16Current/1 -> ComputeDutyCycle/8(sim_au16Current)
  SelectedProfile/1 -> TF_G_111 step2/1, TF_G_112/1, TF_G_111 step1/1
  [A2] -> Relational Operator/1
  Constant8/1 -> Relational Operator/2
  [A4] -> Logical Operator/1
  Relational Operator/1 -> Logical Operator/2
  Logical Operator/1 -> Data Type Conversion2/1
  Data Type Conversion2/1 -> If/1
